simulink model "EV_VehicleLevel_Architecture"  (R2025b)
settings: Solver=VariableStepAuto  StartTime=0.0  StopTime=10.0  RelTol=1e-3
settings Model: DataDictionary=systemParams.sldd  Creator=smuckati  LastModifiedBy=smuckati
settings OptimizationCC: UseDivisionForNetSlopeComputation=on
settings RTWCC: GPUComputeCapability=3.5

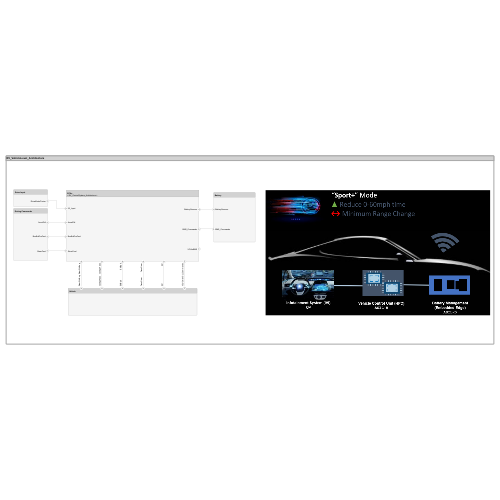
[thumbnail: Simulink's stored preview of the top-level diagram]
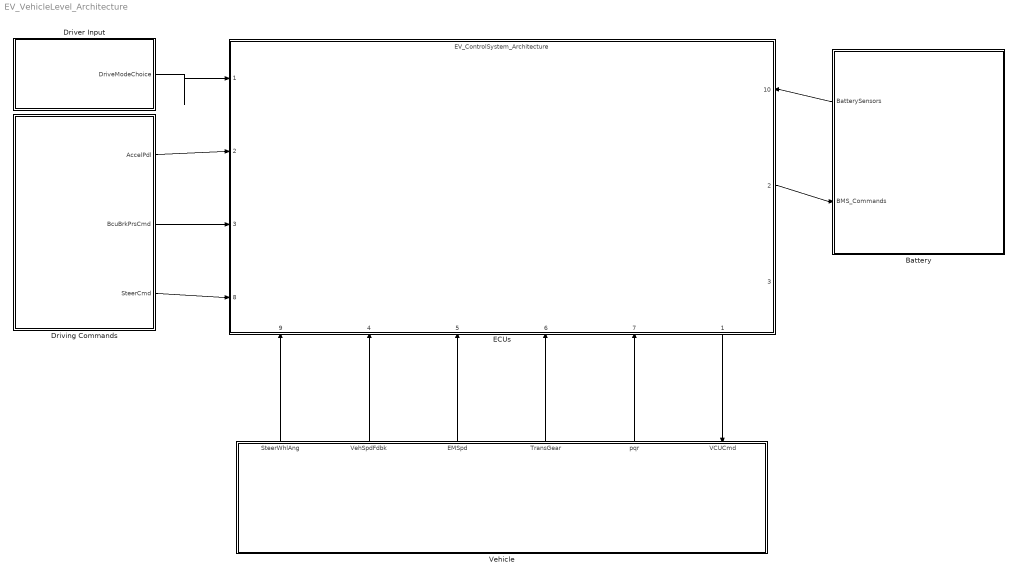
== system EV_VehicleLevel_Architecture ==
  Battery : Subsystem
      settings: PortSchema="{\"entries\":[{\"content\":{\"headerSize\":26,\"margin\":15,\"minimumSpacing\":25,\"sides\":[{\"content\":{\"connectorIds\":[\"Out1\",\"In1\"]},\"type\":\"ConnectorPlacement.EquallySpacedRectSide\",\"uuid\":\"0bbc9e3d-7235-47d6-ad6f-dd1f8eb5ef8f\"},{\"content\":{\"side\":\"RIGHT\"},\"type\":\"ConnectorPlacement.EquallySpacedRectSide\",\"uuid\":\"65cf6885-6ff6-4737-9f0f-48431dc9ec05\"},{\"content\":{\"side\":\"TOP\"},\"type\":\"ConnectorPlacement.EquallySpacedRectSide\",\"uuid\":\"345e4547-f67c-4bab-8588-ce41d45f9363\"}]},\"type\":\"ConnectorPlacement.EquallySpacedConnector\",\"uuid\":\"b8001fcd-770d-4504-9144-d19717d53d24\"}],\"packageUris\":[\"http://schema.mathworks.com/mf0/Connector/R2020b\"],\"version\":\"1.0\"}"
  Driver Input : Subsystem
      settings: PortSchema="{\"entries\":[{\"content\":{\"headerSize\":26,\"margin\":15,\"minimumSpacing\":25,\"sides\":[{\"content\":{},\"type\":\"ConnectorPlacement.EquallySpacedRectSide\",\"uuid\":\"0bbc9e3d-7235-47d6-ad6f-dd1f8eb5ef8f\"},{\"content\":{\"connectorIds\":[\"Out1\"],\"side\":\"RIGHT\"},\"type\":\"ConnectorPlacement.EquallySpacedRectSide\",\"uuid\":\"65cf6885-6ff6-4737-9f0f-48431dc9ec05\"},{\"content\":{\"side\":\"TOP\"},\"type\":\"ConnectorPlacement.EquallySpacedRectSide\",\"uuid\":\"345e4547-f67c-4bab-8588-ce41d45f9363\"}]},\"type\":\"ConnectorPlacement.EquallySpacedConnector\",\"uuid\":\"b8001fcd-770d-4504-9144-d19717d53d24\"}],\"packageUris\":[\"http://schema.mathworks.com/mf0/Connector/R2020b\"],\"version\":\"1.0\"}"
  Driving Commands : Subsystem
      settings: PortSchema="{\"entries\":[{\"content\":{\"headerSize\":26,\"margin\":15,\"minimumSpacing\":25,\"sides\":[{\"content\":{},\"type\":\"ConnectorPlacement.EquallySpacedRectSide\",\"uuid\":\"0bbc9e3d-7235-47d6-ad6f-dd1f8eb5ef8f\"},{\"content\":{\"connectorIds\":[\"Out1\",\"Out2\",\"Out3\"],\"side\":\"RIGHT\"},\"type\":\"ConnectorPlacement.EquallySpacedRectSide\",\"uuid\":\"65cf6885-6ff6-4737-9f0f-48431dc9ec05\"},{\"content\":{\"side\":\"TOP\"},\"type\":\"ConnectorPlacement.EquallySpacedRectSide\",\"uuid\":\"345e4547-f67c-4bab-8588-ce41d45f9363\"}]},\"type\":\"ConnectorPlacement.EquallySpacedConnector\",\"uuid\":\"b8001fcd-770d-4504-9144-d19717d53d24\"}],\"packageUris\":[\"http://schema.mathworks.com/mf0/Connector/R2020b\"],\"version\":\"1.0\"}"
  ECUs : ModelReference  ModelNameDialog=EV_ControlSystem_Architecture.slx  SimulationMode=Normal  ModelReferenceVersion=6.0
      settings: PortSchema="{\"entries\":[{\"content\":{\"headerSize\":38,\"margin\":15,\"minimumSpacing\":25,\"sides\":[{\"content\":{\"connectorIds\":[\"In1\",\"In2\",\"In3\",\"In8\"]},\"type\":\"ConnectorPlacement.EquallySpacedRectSide\",\"uuid\":\"64f986c3-d2b0-47bb-a0ac-06ba247e0759\"},{\"content\":{\"connectorIds\":[\"In10\",\"Out2\",\"Out3\"],\"side\":\"RIGHT\"},\"type\":\"ConnectorPlacement.EquallySpacedRectSide\",\"uuid\":\"db6a84b2-8bbf-456f-ab87-de1f9f3ff13a\"},{\"content\":{\"side\":\"TOP\"},\"type\":\"ConnectorPlacement.EquallySpacedRectSide\",\"uuid\":\"fb4ddf26-0453-4a4d-a4b4-5e4833782acf\"},{\"content\":{\"connectorIds\":[\"In9\",\"In4\",\"In5\",\"In6\",\"In7\",\"Out1\"],\"side\":\"BOTTOM\"},\"type\":\"ConnectorPlacement.EquallySpacedRectSide\",\"uuid\":\"d635bb9a-0b6b-4b7f-ab50-e703f751f120\"}]},\"type\":\"ConnectorPlacement.EquallySpacedConnector\",\"uuid\":\"9b897f9e-5ccd-4129-9810-7c583501cf37\"}],\"packageUris\":[\"http://schema.mathworks.com/mf0/Connector/R2020b\"],\"version\":\"1.0\"}"
  Vehicle : Subsystem
      settings: PortSchema="{\"entries\":[{\"content\":{\"headerSize\":26,\"margin\":15,\"minimumSpacing\":25,\"sides\":[{\"content\":{},\"type\":\"ConnectorPlacement.EquallySpacedRectSide\",\"uuid\":\"0bbc9e3d-7235-47d6-ad6f-dd1f8eb5ef8f\"},{\"content\":{\"side\":\"RIGHT\"},\"type\":\"ConnectorPlacement.EquallySpacedRectSide\",\"uuid\":\"65cf6885-6ff6-4737-9f0f-48431dc9ec05\"},{\"content\":{\"connectorIds\":[\"Out4\",\"Out1\",\"Out2\",\"Out3\",\"Out5\",\"In1\"],\"side\":\"TOP\"},\"type\":\"ConnectorPlacement.EquallySpacedRectSide\",\"uuid\":\"345e4547-f67c-4bab-8588-ce41d45f9363\"}]},\"type\":\"ConnectorPlacement.EquallySpacedConnector\",\"uuid\":\"b8001fcd-770d-4504-9144-d19717d53d24\"}],\"packageUris\":[\"http://schema.mathworks.com/mf0/Connector/R2020b\"],\"version\":\"1.0\"}"
  wires:
  ECUs/2 -> Battery/1(BMS_Commands)
  ECUs/1 -> Vehicle/1(VCUCmd)
  Driving Commands/1(AccelPdl) -> ECUs/2
  Driving Commands/2(BcuBrkPrsCmd) -> ECUs/3
  Battery/1(BatterySensors) -> ECUs/10
  Vehicle/5(pqr) -> ECUs/7
  Vehicle/3(TransGear) -> ECUs/6
  Vehicle/1(VehSpdFdbk) -> ECUs/4
  Vehicle/2(EMSpd) -> ECUs/5
  Vehicle/4(SteerWhlAng) -> ECUs/9
  Driving Commands/3(SteerCmd) -> ECUs/8
  Driver Input/1(DriveModeChoice) -> ECUs/1

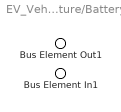
== system EV_VehicleLevel_Architecture/Battery ==
  Bus Element In1 : Inport  PortName=BMS_Commands
  Bus Element Out1 : Outport  PortName=BatterySensors

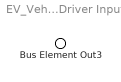
== system EV_VehicleLevel_Architecture/Driver Input ==
  Bus Element Out3 : Outport  PortName=DriveModeChoice

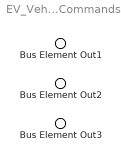
== system EV_VehicleLevel_Architecture/Driving Commands ==
  Bus Element Out1 : Outport  PortName=AccelPdl
  Bus Element Out2 : Outport  Port=2  PortName=BcuBrkPrsCmd
  Bus Element Out3 : Outport  Port=3  PortName=SteerCmd

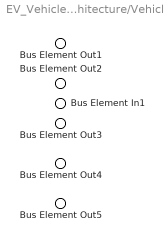
== system EV_VehicleLevel_Architecture/Vehicle ==
  Bus Element In1 : Inport  PortName=VCUCmd
  Bus Element Out1 : Outport  PortName=VehSpdFdbk
  Bus Element Out2 : Outport  Port=2  PortName=EMSpd
  Bus Element Out3 : Outport  Port=3  PortName=TransGear
  Bus Element Out4 : Outport  Port=4  PortName=SteerWhlAng
  Bus Element Out5 : Outport  Port=5  PortName=pqr
